simulink model "serialDemo_test"  (R2023a)
settings: Solver=FixedStepAuto  StartTime=0.0  StopTime=10.0  FixedStep=1e-3  RelTol=1e-3  EnableMultiTasking=on
libraries: frdmk64flib x5, etargetslib x2
settings Model: ExtModeTrigDuration=5  Creator=joell  LastModifiedBy=joell
settings SolverCC: AlgebraicLoopSolver=TrustRegion  AutoInsertRateTranBlk=on
settings DataIOCC: LimitDataPoints=on
settings OptimizationCC: EnhancedBackFolding=on  PassReuseOutputArgsAs=Individual arguments  ZeroExternalMemoryAtStartup=off  ZeroInternalMemoryAtStartup=off  MaxStackSize=64  OptimizeBlockOrder=speed  DifferentSizesBufferReuse=on  OptimizationCustomize=off  EfficientTunableParamExpr=on
settings DebuggingCC: ParameterTunabilityLossMsg=error  UnconnectedInputMsg=warning  UnconnectedOutputMsg=warning  UnconnectedLineMsg=warning  AllowSymbolicDim=off  SFUnexpectedBacktrackingDiag=warning  SFNoUnconditionalDefaultTransitionDiag=warning  SFExecutionAtInitializationDiag=none  ArithmeticOperatorsInVariantConditions=warning
settings HardwareCC: ProdBitPerPointer=32  ProdBitPerSizeT=32  ProdBitPerPtrDiffT=32  ProdLargestAtomicInteger=Long  ProdLargestAtomicFloat=Double  ProdWordSize=32  ProdHWDeviceType=ARM Compatible->ARM Cortex
settings ModelReferenceCC: EnableRefExpFcnMdlSchedulingChecks=on
settings SFSimCC: SimUseLocalCustomCode=off  MATLABDynamicMemAlloc=off  CustomCodeUndefinedFunction=UseInterfaceOnly
settings RTWCC: Description=Embedded Coder  SystemTargetFile=ert.tlc  HardwareBoard=NXP FRDM-K64F  TLCOptions="-aInlineSetEventsForThisBaseRateFcn=TLC_FALSE -aSuppressMultiTaskScheduler=TLC_FALSE  -aRateBasedStepFcn=0"  TemplateMakefile=ert_default_tmf  RTWUseLocalCustomCode=off  Toolchain=GNU Tools for ARM Embedded Processors  DLArmComputeVersion=19.05
settings CodeAppCC: ForceParamTrailComments=on  IgnoreCustomStorageClasses=off  OperatorAnnotations=on  SimulinkDataObjDesc=on  SFDataObjDesc=on  InsertBlockDesc=on
settings ERTTargetCC: ExtModeTransport=4  ExtModeMexFile=sendToCommService
settings ConfigComp: CovMetricSettings=dw  CovSaveCumulativeToWorkspaceVar=on  CovSaveSingleToWorkspaceVar=on  CovExternalEMLEnable=off  CovSFcnEnable=off

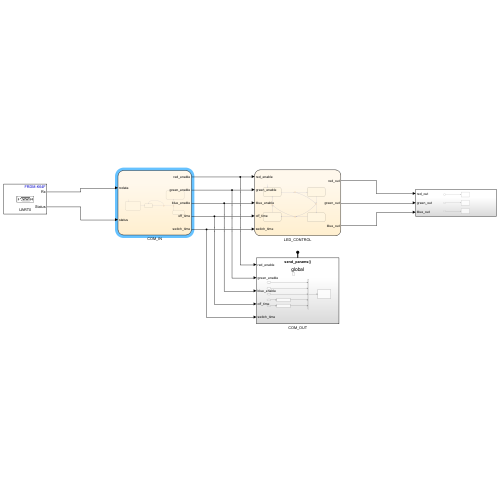
[thumbnail: Simulink's stored preview of the top-level diagram]
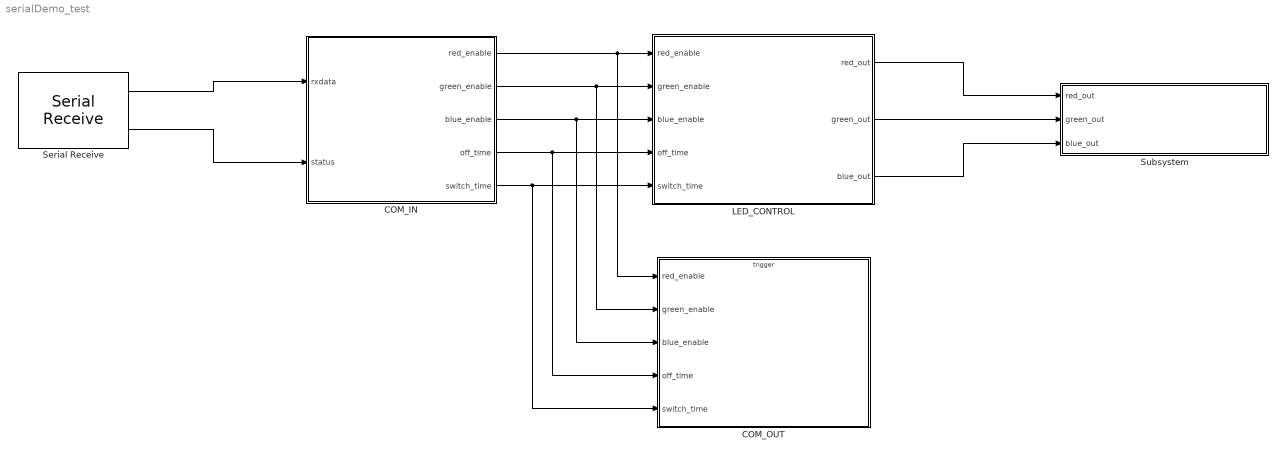
== system serialDemo_test ==
  COM_IN : Stateflow chart  TreatAsAtomicUnit=on
  COM_OUT : Subsystem  TreatAsAtomicUnit=on
  LED_CONTROL : Stateflow chart  TreatAsAtomicUnit=on
      settings: PortSchema="{\"entries\":[{\"content\":{\"sides\":[{\"content\":{\"connectorIds\":[\"In2\",\"In5\",\"In4\",\"In1\",\"In3\"]},\"type\":\"ConnectorPlacement.EquallySpacedRectSide\",\"uuid\":\"927ca74e-c033-4f6d-85ad-003e30104f68\"},{\"content\":{\"connectorIds\":[\"Out3\",\"Out2\",\"Out1\"],\"side\":\"RIGHT\"},\"type\":\"ConnectorPlacement.EquallySpacedRectSide\",\"uuid\":\"9965330c-7990-4e14-9c34-766c1f65c963\"},{\"content\":{\"side\":\"TOP\"},\"type\":\"ConnectorPlacement.EquallySpacedRectSide\",\"uuid\":\"99f9e81e-4521-4a19-ab83-21d6f885dfed\"}]},\"type\":\"ConnectorPlacement.EquallySpacedConnector\",\"uuid\":\"6b0ef790-2846-4154-b672-ecc98352102f\"}],\"packageUris\":[\"http://schema.mathworks.com/mf0/Connector/R2020b\"],\"version\":\"1.0\"}"
  Serial Receive : frdmk64flib/Serial Receive  SCIModule=0  Baudrate=uint32(9600)  Parity=None  StopBits=1  HardwareFlowControl=None  ByteOrder=LittleEndian  DataType=uint8  DataLength=10  BlockingMode=off  OutputStatus=on  SampleTime=0.1
  Subsystem : Subsystem
  wires:
  Serial Receive/1 -> COM_IN/1(rxdata)
  Serial Receive/2 -> COM_IN/2(status)
  COM_IN/1(red_enable) -> COM_OUT/1(red_enable), LED_CONTROL/2(red_enable)
  COM_IN/2(green_enable) -> COM_OUT/2(green_enable), LED_CONTROL/5(green_enable)
  COM_IN/3(blue_enable) -> COM_OUT/3(blue_enable), LED_CONTROL/4(blue_enable)
  COM_IN/4(off_time) -> COM_OUT/4(off_time), LED_CONTROL/1(off_time)
  COM_IN/5(switch_time) -> COM_OUT/5(switch_time), LED_CONTROL/3(switch_time)
  LED_CONTROL/3(red_out) -> Subsystem/1(red_out)
  LED_CONTROL/2(green_out) -> Subsystem/2(green_out)
  LED_CONTROL/1(blue_out) -> Subsystem/3(blue_out)

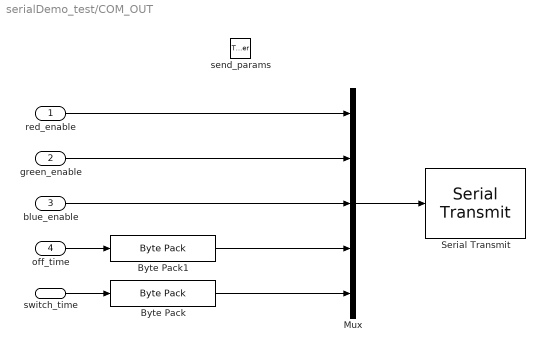
== system serialDemo_test/COM_OUT ==
  red_enable : Inport  OutDataTypeStr=uint8
  green_enable : Inport  Port=2  OutDataTypeStr=uint8
  blue_enable : Inport  Port=3  OutDataTypeStr=uint8
  off_time : Inport  Port=4  OutDataTypeStr=single
  switch_time : Inport  Port=5  OutDataTypeStr=uint16
  send_params : TriggerPort  TriggerType=function-call  IsSimulinkFunction=on  FunctionName=send_params  VariantControl=(inherit)
  Byte Pack : etargetslib/Byte Pack  datatypes={'uint16'}  byteAlign=1
  Byte Pack1 : etargetslib/Byte Pack  datatypes={'single'}  byteAlign=1
  Mux : Mux  Inputs=5
  Serial Transmit : frdmk64flib/Serial Transmit  SCIModule=0  Baudrate=uint32(9600)  Parity=None  StopBits=1  HardwareFlowControl=None  ByteOrder=LittleEndian  BlockingMode=on  OutputStatus=off
  wires:
  red_enable/1 -> Mux/1
  green_enable/1 -> Mux/2
  blue_enable/1 -> Mux/3
  off_time/1 -> Byte Pack1/1
  Byte Pack1/1 -> Mux/4
  switch_time/1 -> Byte Pack/1
  Byte Pack/1 -> Mux/5
  Mux/1 -> Serial Transmit/1

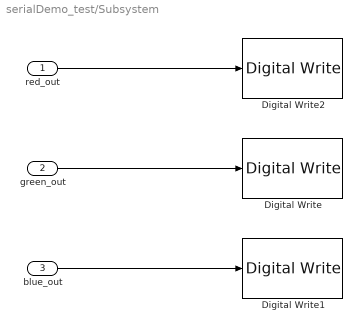
== system serialDemo_test/Subsystem ==
  red_out : Inport  OutDataTypeStr=uint8
  green_out : Inport  Port=2  OutDataTypeStr=uint8
  blue_out : Inport  Port=3  OutDataTypeStr=uint8
  Digital Write : frdmk64flib/Digital Write  Whichpin=GREEN_LED
  Digital Write1 : frdmk64flib/Digital Write  Whichpin=BLUE_LED
  Digital Write2 : frdmk64flib/Digital Write  Whichpin=RED_LED
  wires:
  red_out/1 -> Digital Write2/1
  green_out/1 -> Digital Write/1
  blue_out/1 -> Digital Write1/1

== stateflow chart serialDemo_test/LED_CONTROL ==
  state RED_ON
    entry:
    red_out = 1;
    green_out = 0;
    blue_out = 0;
  state OFF
    entry:
    red_out = 0;
    green_out = 0;
    blue_out = 0;
  state BLUE_OFF
    entry:
    red_out = 0;
    green_out = 0;
    blue_out = 1;
  state GREEN_ON
    entry:
    red_out = 0;
    green_out = 1;
    blue_out = 0;
  (default) -> OFF
  OFF -> (junction 3) : after(off_time,sec)
  (junction 3) -> RED_ON [order 1] : [red_enable==1]
  (junction 3) -> (junction 6) [order 2]
  (junction 8) -> OFF
  RED_ON -> (junction 6) : after(switch_time, msec)
  (junction 6) -> (junction 7) [order 2]
  (junction 6) -> GREEN_ON [order 1] : [green_enable == 1]
  (junction 7) -> (junction 8) [order 2]
  BLUE_OFF -> (junction 8) : after(switch_time, msec)
  (junction 7) -> BLUE_OFF [order 1] : [blue_enable == 1]
  GREEN_ON -> (junction 7) : after(switch_time, msec)
  data: off_time input single; red_enable input uint8; switch_time input uint16; blue_out output uint8; green_out output uint8; red_out output uint8; blue_enable input uint8; green_enable input uint8

== stateflow chart serialDemo_test/COM_IN ==
  settings: executeAtInitialization=1
  state SET_PARAM
    entry:
    red_enable = rxdata(3);
    green_enable = rxdata(4);
    blue_enable = rxdata(5);
    off_time = typecast(rxdata(6:9), 'single');
    switch_time = typecast(rxdata(10:11), 'uint16');
  state INITIAL
    % Set the initial values of parameters
    entry:
    red_enable = 1;
    green_enable = 1;
    blue_enable = 1;
    off_time = 0.5; % In Seconds
    switch_time = 200; % In Milliseconds
  state STANDBY
    % Waiting for COM
  state ECHO_PARAM
    entry:
    send_params();
  (junction 13) -> SET_PARAM [order 1] : [rxdata(2) == hex2dec('55')]
  (default) -> INITIAL
  (junction 10) -> STANDBY [order 2]
  INITIAL -> STANDBY
  STANDBY -> (junction 10) : [status == 0]
  (junction 10) -> (junction 13) [order 1] : [rxdata(1) == hex2dec('16')]
  (junction 13) -> ECHO_PARAM [order 2] : [rxdata(2)==hex2dec('22')]
  data: red_enable output uint8; green_enable output uint8; blue_enable output uint8; off_time output single; switch_time output uint16; rxdata input uint8; status input uint8
